simulink model "Noa_Nofusion_backup"  (R2020b)
settings: Solver=FixedStepDiscrete  StartTime=0.0  StopTime=Inf  FixedStep=0.02  RelTol=1e-3
PostLoadFcn:
  | if any(exist('dsrtsu_mdlpostloadfcn', 'file') ~= 0), dsrtsu_mdlpostloadfcn('Execute', bdroot); end
InitFcn:
  | , if any(exist('rtifpga_mdlclblib', 'file') ~= 0), rtifpga_mdlclblib('Init', bdroot); end,
  | , if any(exist('dsmpb_private', 'file') ~= 0), dsmpb_private('dsmpb_mdlclblib', 'Init', bdroot); end,
undefined symbols (not defined in the file): ACC_TimeGap_DecSetSwt, ACC_TimeGap_IncSetSwt, AccelPedalPosn, AccelPedalPosnVldty, AccelPedlPosnDiagc, AccPedalOverride, ACU_ShiftInProgress, ADAS_Posn_CurLane, AESSwtReq, ALC_SwtReq, BrkPedalSts, CC_ACC_CANCEL_OFFSwt, CC_ACC_CRUISE_OFFSwt, CC_ACC_DecSetSpd_SetSwt, CC_ACC_IncSetSpd_ResuSwt, CC_ACCSwtErr, CharSpd_ms, CSA_NODE, CURRENT_GEAR, CurrentGearValid, DiscIntNeverNeededParam, DrvDoorSts, DrvSBR, DrvTrqReqOvld, ECMACCInterface, ECMRespACC, ELKSwtReq, EngLimpHomeSts, EngSpd, EngState, EngState_PHEV, EngTrqMaxActSpd, EngTrqMinAct, EPS_DrvInpTrqVal_HighReslolution, EPS_FailSts, EPS_LKATorqOvrlDlvd, EPS_LKATorqOvrlDlvdVld, EPS_LKATrqOvlDlvdSts, EPS_SteerMod, EPS_TrqSnsrSts, EQ4_APPINFO, EQ4_LA_ELEM, EQ4_LA_HDR, EQ4_LAP_ELEM, EQ4_LAP_HDR, EQ4_LH_ELEM, EQ4_LH_HDR, EQ4_LRE_ELEM, EQ4_LRE_HDR, ESS_PedSwtReq, ESS_VehSwtReq, FFogLmpSts_F_Pbox, FLWheelDriveDirection, FLWheelSpd, FrntWiprSwtSts, FrntWshrSwtSts, FRWheelDriveDirection, FRWheelSpd, HazardLmpSwtSts, HCU_AccelPedalPosn_Diag ... (+152)
libraries: simulink x117, dsmpblib x30
(part 8 of 11)

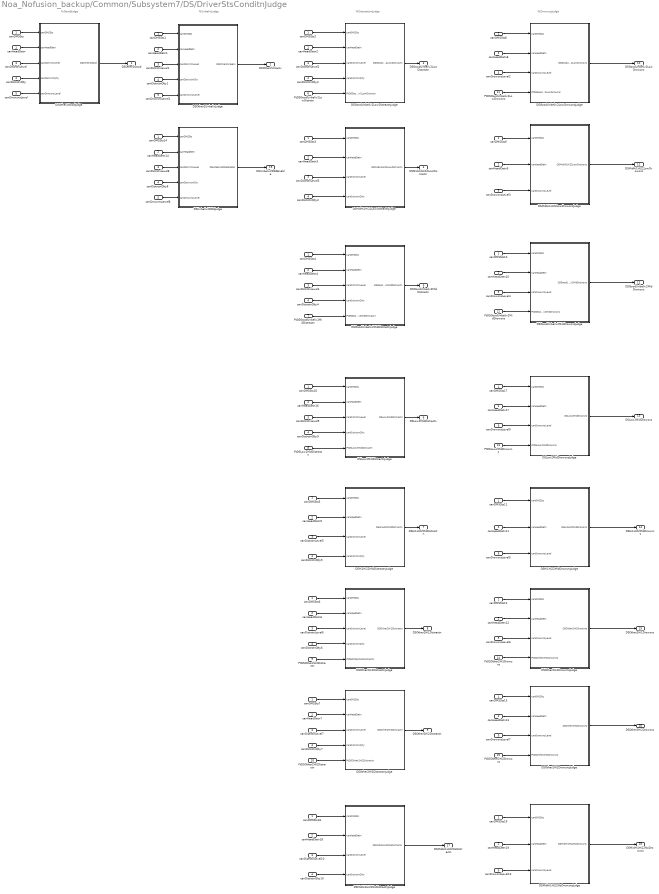
== system Noa_Nofusion_backup/Common/Subsystem7/DS/DriverStsConditnJudge ==
  note: %GoodJudge
  note: %UnbelivJudge
  note: %DistractionJudge
  note: %DrowsnsJudge
  canDMSSts : Inport
  canHeadDetn : Inport  Port=2
  canDistrctnLevel : Inport  Port=3
  canDistrctnQlty : Inport  Port=4
  canDrowsnsLevel : Inport  Port=5
  PtDSGoodUnbeliv2LowDistrctn : Inport  Port=6
  PtDSGoodUnbeliv2MidDistractn : Inport  Port=7
  PtDSLow2MidDistractn : Inport  Port=8
  PtDSOther2Hi1Distractn : Inport  Port=9
  PtDSOther2Hi2Distractn : Inport  Port=10
  PtDSGoodUnbeliv2LowDrowsns : Inport  Port=11
  PtDSGoodUnbeliv2MidDrowsns : Inport  Port=12
  PtDSLow2MidDrowsns : Inport  Port=13
  PtDSOther2Hi1Drowsns : Inport  Port=14
  PtDSOther2Hi2Drowsns : Inport  Port=15
  DSGoodUnbeliv2LowDistractnJudge : Subsystem
  DSGoodUnbeliv2LowDrowsnsJudge : Subsystem
  DSGoodUnbeliv2MidDistractnJudge : Subsystem
  DSGoodUnbeliv2MidDrowsnsJudge : Subsystem
  DSHi1Hi22MidDistractnJudge : Subsystem
  DSHi1Hi22MidDrowsnsJudge : Subsystem
  DSLow2MidDistractnJudge : Subsystem
  DSLow2MidDrowsnsJudge : Subsystem
  DSMidHi1Hi22LowDistractnJudge : Subsystem
  DSMidHi1Hi22LowDrowsnsJudge : Subsystem
  DSMidHi1Hi22NoDistractnJudge : Subsystem
  DSMidHi1Hi22NoDrowsnsJudge : Subsystem
  DSOther2GoodJudge : Subsystem
  DSOther2Hi1DistractnJudge : Subsystem
  DSOther2Hi1DrowsnsJudge : Subsystem
  DSOther2Hi2DistractnJudge : Subsystem
  DSOther2Hi2DrowsnsJudge : Subsystem
  DSOther2UnbelivJudge : Subsystem
  DSUnbeliv2DDAJudge : Subsystem
  canDMSSts{1..14,16..19} (18 alike) : InportShadow
  canDistrctnLevel{1..10} (10 alike) : InportShadow  Port=3
  canDistrctnQlty{1..10} (10 alike) : InportShadow  Port=4
  canDrowsnsLevel{1..10} (10 alike) : InportShadow  Port=5
  canHeadDetn{1..14,16..19} (18 alike) : InportShadow  Port=2
  DSOther2Good : Outport
  DSOther2Unbeliv : Outport  Port=2
  DSGoodUnbeliv2LowDistractn : Outport  Port=3
  DSMidHi1Hi22LowDistractn : Outport  Port=4
  DSGoodUnbeliv2MidDistractn : Outport  Port=5
  DSLow2MidDistractn : Outport  Port=6
  DSHi1Hi22MidDistractn : Outport  Port=7
  DSOther2Hi1Distractn : Outport  Port=8
  DSOther2Hi2Distractn : Outport  Port=9
  DSGoodUnbeliv2LowDrowsns : Outport  Port=10
  DSMidHi1Hi22LowDrowsns : Outport  Port=11
  DSGoodUnbeliv2MidDrowsns : Outport  Port=12
  DSLow2MidDrowsns : Outport  Port=13
  DSHi1Hi22MidDrowsns : Outport  Port=14
  DSOther2Hi1Drowsns : Outport  Port=15
  DSOther2Hi2Drowsns : Outport  Port=16
  DSMidHi1Hi22NoDistractn : Outport  Port=17
  DSMidHi1Hi22NoDrowsns : Outport  Port=18
  DSUnbeliv2DDAEnable : Outport  Port=19
  wires:
  canDMSSts/1 -> DSOther2GoodJudge/1(canDMSSts)
  DSOther2GoodJudge/1(DSOther2Good) -> DSOther2Good/1
  canHeadDetn/1 -> DSOther2GoodJudge/2(canHeadDetn)
  canDistrctnLevel/1 -> DSOther2GoodJudge/3(canDistrctnLevel)
  canDistrctnQlty/1 -> DSOther2GoodJudge/4(canDistrctnQlty)
  canDrowsnsLevel/1 -> DSOther2GoodJudge/5(canDrowsnsLevel)
  canDMSSts1/1 -> DSOther2UnbelivJudge/1(canDMSSts)
  canHeadDetn1/1 -> DSOther2UnbelivJudge/2(canHeadDetn)
  canDistrctnLevel1/1 -> DSOther2UnbelivJudge/3(canDistrctnLevel)
  canDistrctnQlty1/1 -> DSOther2UnbelivJudge/4(canDistrctnQlty)
  canDrowsnsLevel1/1 -> DSOther2UnbelivJudge/5(canDrowsnsLevel)
  DSOther2UnbelivJudge/1(DSOther2Unbeliv) -> DSOther2Unbeliv/1
  DSGoodUnbeliv2LowDistractnJudge/1(DSGoodUnbeliv2LowDistractn) -> DSGoodUnbeliv2LowDistractn/1
  canDMSSts2/1 -> DSGoodUnbeliv2LowDistractnJudge/1(canDMSSts)
  canHeadDetn2/1 -> DSGoodUnbeliv2LowDistractnJudge/2(canHeadDetn)
  canDistrctnLevel2/1 -> DSGoodUnbeliv2LowDistractnJudge/3(canDistrctnLevel)
  canDistrctnQlty2/1 -> DSGoodUnbeliv2LowDistractnJudge/4(canDistrctnQlty)
  canDMSSts3/1 -> DSMidHi1Hi22LowDistractnJudge/1(canDMSSts)
  canHeadDetn3/1 -> DSMidHi1Hi22LowDistractnJudge/2(canHeadDetn)
  canDistrctnLevel3/1 -> DSMidHi1Hi22LowDistractnJudge/3(canDistrctnLevel)
  canDistrctnQlty3/1 -> DSMidHi1Hi22LowDistractnJudge/4(canDistrctnQlty)
  DSMidHi1Hi22LowDistractnJudge/1(DSMidHi1Hi22LowDistractn) -> DSMidHi1Hi22LowDistractn/1
  canDMSSts4/1 -> DSGoodUnbeliv2MidDistractnJudge/1(canDMSSts)
  canHeadDetn4/1 -> DSGoodUnbeliv2MidDistractnJudge/2(canHeadDetn)
  canDistrctnLevel4/1 -> DSGoodUnbeliv2MidDistractnJudge/3(canDistrctnLevel)
  canDistrctnQlty4/1 -> DSGoodUnbeliv2MidDistractnJudge/4(canDistrctnQlty)
  DSGoodUnbeliv2MidDistractnJudge/1(DSGoodUnbeliv2MidDistractn) -> DSGoodUnbeliv2MidDistractn/1
  canDMSSts5/1 -> DSHi1Hi22MidDistractnJudge/1(canDMSSts)
  canHeadDetn5/1 -> DSHi1Hi22MidDistractnJudge/2(canHeadDetn)
  canDistrctnLevel5/1 -> DSHi1Hi22MidDistractnJudge/3(canDistrctnLevel)
  canDistrctnQlty5/1 -> DSHi1Hi22MidDistractnJudge/4(canDistrctnQlty)
  DSHi1Hi22MidDistractnJudge/1(DSHi1Hi22MidDistractn) -> DSHi1Hi22MidDistractn/1
  DSOther2Hi1DistractnJudge/1(DSOther2Hi1Distractn) -> DSOther2Hi1Distractn/1
  canDMSSts6/1 -> DSOther2Hi1DistractnJudge/1(canDMSSts)
  canHeadDetn6/1 -> DSOther2Hi1DistractnJudge/2(canHeadDetn)
  canDistrctnLevel6/1 -> DSOther2Hi1DistractnJudge/3(canDistrctnLevel)
  canDistrctnQlty6/1 -> DSOther2Hi1DistractnJudge/4(canDistrctnQlty)
  DSOther2Hi2DistractnJudge/1(DSOther2Hi2Distractn) -> DSOther2Hi2Distractn/1
  canDMSSts7/1 -> DSOther2Hi2DistractnJudge/1(canDMSSts)
  canHeadDetn7/1 -> DSOther2Hi2DistractnJudge/2(canHeadDetn)
  canDistrctnLevel7/1 -> DSOther2Hi2DistractnJudge/3(canDistrctnLevel)
  canDistrctnQlty7/1 -> DSOther2Hi2DistractnJudge/4(canDistrctnQlty)
  DSGoodUnbeliv2LowDrowsnsJudge/1(DSGoodUnbeliv2LowDrowsns) -> DSGoodUnbeliv2LowDrowsns/1
  canDMSSts8/1 -> DSGoodUnbeliv2LowDrowsnsJudge/1(canDMSSts)
  canHeadDetn8/1 -> DSGoodUnbeliv2LowDrowsnsJudge/2(canHeadDetn)
  canDrowsnsLevel2/1 -> DSGoodUnbeliv2LowDrowsnsJudge/3(canDrowsnsLevel)
  DSMidHi1Hi22LowDrowsnsJudge/1(DSMidHi1Hi22LowDrowsns) -> DSMidHi1Hi22LowDrowsns/1
  canDMSSts9/1 -> DSMidHi1Hi22LowDrowsnsJudge/1(canDMSSts)
  canHeadDetn9/1 -> DSMidHi1Hi22LowDrowsnsJudge/2(canHeadDetn)
  canDrowsnsLevel3/1 -> DSMidHi1Hi22LowDrowsnsJudge/3(canDrowsnsLevel)
  canDMSSts10/1 -> DSGoodUnbeliv2MidDrowsnsJudge/1(canDMSSts)
  canHeadDetn10/1 -> DSGoodUnbeliv2MidDrowsnsJudge/2(canHeadDetn)
  canDrowsnsLevel4/1 -> DSGoodUnbeliv2MidDrowsnsJudge/3(canDrowsnsLevel)
  DSGoodUnbeliv2MidDrowsnsJudge/1(DSGoodUnbeliv2MidDrowsns) -> DSGoodUnbeliv2MidDrowsns/1
  DSHi1Hi22MidDrowsnsJudge/1(DSHi1Hi22MidDrowsns) -> DSHi1Hi22MidDrowsns/1
  canDrowsnsLevel5/1 -> DSHi1Hi22MidDrowsnsJudge/3(canDrowsnsLevel)
  canHeadDetn11/1 -> DSHi1Hi22MidDrowsnsJudge/2(canHeadDetn)
  canDMSSts11/1 -> DSHi1Hi22MidDrowsnsJudge/1(canDMSSts)
  canDMSSts12/1 -> DSOther2Hi1DrowsnsJudge/1(canDMSSts)
  canHeadDetn12/1 -> DSOther2Hi1DrowsnsJudge/2(canHeadDetn)
  canDrowsnsLevel6/1 -> DSOther2Hi1DrowsnsJudge/3(canDrowsnsLevel)
  DSOther2Hi1DrowsnsJudge/1(DSOther2Hi1Drowsns) -> DSOther2Hi1Drowsns/1
  canDrowsnsLevel7/1 -> DSOther2Hi2DrowsnsJudge/3(canDrowsnsLevel)
  canHeadDetn13/1 -> DSOther2Hi2DrowsnsJudge/2(canHeadDetn)
  canDMSSts13/1 -> DSOther2Hi2DrowsnsJudge/1(canDMSSts)
  DSOther2Hi2DrowsnsJudge/1(DSOther2Hi2Drowsns) -> DSOther2Hi2Drowsns/1
  DSLow2MidDistractnJudge/1(DSLow2MidDistractn) -> DSLow2MidDistractn/1
  canDistrctnQlty9/1 -> DSLow2MidDistractnJudge/4(canDistrctnQlty)
  canDistrctnLevel9/1 -> DSLow2MidDistractnJudge/3(canDistrctnLevel)
  canHeadDetn16/1 -> DSLow2MidDistractnJudge/2(canHeadDetn)
  canDMSSts16/1 -> DSLow2MidDistractnJudge/1(canDMSSts)
  canDrowsnsLevel9/1 -> DSLow2MidDrowsnsJudge/3(canDrowsnsLevel)
  canHeadDetn17/1 -> DSLow2MidDrowsnsJudge/2(canHeadDetn)
  canDMSSts17/1 -> DSLow2MidDrowsnsJudge/1(canDMSSts)
  DSLow2MidDrowsnsJudge/1(DSLow2MidDrowsns) -> DSLow2MidDrowsns/1
  canDistrctnQlty10/1 -> DSMidHi1Hi22NoDistractnJudge/4(canDistrctnQlty)
  canDistrctnLevel10/1 -> DSMidHi1Hi22NoDistractnJudge/3(canDistrctnLevel)
  canHeadDetn18/1 -> DSMidHi1Hi22NoDistractnJudge/2(canHeadDetn)
  canDMSSts18/1 -> DSMidHi1Hi22NoDistractnJudge/1(canDMSSts)
  DSMidHi1Hi22NoDistractnJudge/1(DSMidHi1Hi22NoDistractn) -> DSMidHi1Hi22NoDistractn/1
  canDrowsnsLevel10/1 -> DSMidHi1Hi22NoDrowsnsJudge/3(canDrowsnsLevel)
  canHeadDetn19/1 -> DSMidHi1Hi22NoDrowsnsJudge/2(canHeadDetn)
  canDMSSts19/1 -> DSMidHi1Hi22NoDrowsnsJudge/1(canDMSSts)
  DSMidHi1Hi22NoDrowsnsJudge/1(DSMidHi1Hi22NoDrowsns) -> DSMidHi1Hi22NoDrowsns/1
  canDrowsnsLevel8/1 -> DSUnbeliv2DDAJudge/5(canDrowsnsLevel)
  canDistrctnQlty8/1 -> DSUnbeliv2DDAJudge/4(canDistrctnQlty)
  canDistrctnLevel8/1 -> DSUnbeliv2DDAJudge/3(canDistrctnLevel)
  canHeadDetn14/1 -> DSUnbeliv2DDAJudge/2(canHeadDetn)
  canDMSSts14/1 -> DSUnbeliv2DDAJudge/1(canDMSSts)
  DSUnbeliv2DDAJudge/1(DSUnbeliv2DDAEnable) -> DSUnbeliv2DDAEnable/1
  PtDSGoodUnbeliv2LowDistrctn/1 -> DSGoodUnbeliv2LowDistractnJudge/5(PtDSGoodUnbeliv2LowDistrctn)
  PtDSGoodUnbeliv2MidDistractn/1 -> DSGoodUnbeliv2MidDistractnJudge/5(PtDSGoodUnbeliv2MidDistractn)
  PtDSLow2MidDistractn/1 -> DSLow2MidDistractnJudge/5(PtDSLow2MidDistractn)
  PtDSOther2Hi1Distractn/1 -> DSOther2Hi1DistractnJudge/5(PtDSOther2Hi1Distractn)
  PtDSOther2Hi2Distractn/1 -> DSOther2Hi2DistractnJudge/5(PtDSOther2Hi2Distractn)
  PtDSGoodUnbeliv2LowDrowsns/1 -> DSGoodUnbeliv2LowDrowsnsJudge/4(PtDSGoodUnbeliv2LowDrowsns)
  PtDSGoodUnbeliv2MidDrowsns/1 -> DSGoodUnbeliv2MidDrowsnsJudge/4(PtDSGoodUnbeliv2MidDrowsns)
  PtDSLow2MidDrowsns/1 -> DSLow2MidDrowsnsJudge/4(PtDSLow2MidDrowsns)
  PtDSOther2Hi1Drowsns/1 -> DSOther2Hi1DrowsnsJudge/4(PtDSOther2Hi1Drowsns)
  PtDSOther2Hi2Drowsns/1 -> DSOther2Hi2DrowsnsJudge/4(PtDSOther2Hi2Drowsns)

== system Noa_Nofusion_backup/Subsystem2/ACCOSM/HWA_Task100ms1/OTL1 ==
  vRef : Inport
  tCycle : Inport  Port=2
  tSameHandle : Inport  Port=3
  CutIn : Inport  Port=4
  P0Dx : Inport  Port=5
  P0Dy : Inport  Port=6
  EgoDDeltaX : Inport  Port=7
  EgoDDeltaY : Inport  Port=8
  EgoCosOfPsi : Inport  Port=9
  EgoSinOfPsi : Inport  Port=10
  Memory31 : Memory  InitialCondition=zeros(24,1)  InheritSampleTime=on
  Memory32 : Memory  InitialCondition=zeros(24,1)  InheritSampleTime=on
  Memory33 : Memory  InitialCondition=uint8(0)  InheritSampleTime=on
  P0TrajHistCalc01 : MATLAB Function  TreatAsAtomicUnit=on
  P0TrajHistCalc1 : MATLAB Function  TreatAsAtomicUnit=on
  Terminator : Terminator
  Terminator1 : Terminator
  Terminator2 : Terminator
  LineValid : Outport
  a : Outport  Port=2
  b : Outport  Port=3
  c : Outport  Port=4
  d : Outport  Port=5
  dxMin : Outport  Port=6
  dxMax : Outport  Port=7
  wires:
  vRef/1 -> P0TrajHistCalc01/1(vRef)
  CutIn/1 -> P0TrajHistCalc01/4(CutIn)
  P0TrajHistCalc1/8(d) -> d/1
  P0TrajHistCalc1/10(dxMax) -> dxMax/1
  P0TrajHistCalc1/9(dxMin) -> dxMin/1
  P0TrajHistCalc1/7(c) -> c/1
  P0TrajHistCalc1/6(b) -> b/1
  P0TrajHistCalc1/5(a) -> a/1
  P0TrajHistCalc1/4(LineValid) -> LineValid/1
  P0TrajHistCalc1/3(P0TrajHistDyv) -> Terminator2/1
  P0TrajHistCalc1/2(P0TrajHistDxv) -> Terminator1/1
  P0TrajHistCalc1/1(P0TrajHistNum) -> Terminator/1
  P0Dy/1 -> P0TrajHistCalc01/6(P0Dy)
  P0Dx/1 -> P0TrajHistCalc01/5(P0Dx)
  tSameHandle/1 -> P0TrajHistCalc01/3(tSameHandle)
  EgoCosOfPsi/1 -> P0TrajHistCalc01/9(EgoCosOfPsi)
  tCycle/1 -> P0TrajHistCalc01/2(tCycle)
  Memory31/1 -> P0TrajHistCalc01/13(P0TrajHistDyvK1)
  EgoDDeltaY/1 -> P0TrajHistCalc01/8(EgoDDeltaY)
  P0TrajHistCalc01/2(P0TrajHistDxv) -> Memory32/1, P0TrajHistCalc1/2(P0TrajHistDxv1)
  Memory32/1 -> P0TrajHistCalc01/12(P0TrajHistDxvK1)
  P0TrajHistCalc01/1(P0TrajHistNum) -> Memory33/1, P0TrajHistCalc1/1(P0TrajHistNum1)
  EgoSinOfPsi/1 -> P0TrajHistCalc01/10(EgoSinOfPsi)
  Memory33/1 -> P0TrajHistCalc01/11(P0TrajHistNumK1)
  P0TrajHistCalc01/3(P0TrajHistDyv) -> Memory31/1, P0TrajHistCalc1/3(P0TrajHistDyv1)
  EgoDDeltaX/1 -> P0TrajHistCalc01/7(EgoDDeltaX)

== system Noa_Nofusion_backup/Subsystem2/ACCOSM/HWA_Task100ms1/Trajectory ==
  Kap : Inport
  VxvRef : Inport  Port=2
  AlpSideSlipAngle : Inport  Port=3
  ObjValid : Inport  Port=4
  ObjDx : Inport  Port=5
  ObjDy : Inport  Port=6
  ObjClass : Inport  Port=7
  ObjCntAlive : Inport  Port=8
  Terminator{1,3..10} (9 alike) : Terminator
  Trajectory : Subsystem  mask{ObjNum=15, TrajNum=10, BufNum=24}
      mask prompts: ObjNum "ObjectNumber"; TrajNum "TrajectoryNumber"; BufNum "BufferNumber"
  Out8 : Outport
  Out9 : Outport  Port=2
  Out10 : Outport  Port=3
  Out11 : Outport  Port=4
  Out12 : Outport  Port=5
  Out13 : Outport  Port=6
  EgoMove : Outport  Port=7
  wires:
  Trajectory/16(EgoMove) -> EgoMove/1
  Trajectory/11(TrajHistBufferBValid) -> Out11/1
  Trajectory/12(TrajHistBufferDxv) -> Out12/1
  Trajectory/13(TrajHistBufferDyv) -> Out13/1
  ObjValid/1 -> Trajectory/4(ObjValid)
  ObjDx/1 -> Trajectory/5(ObjectDx)
  ObjDy/1 -> Trajectory/6(ObjectDy)
  ObjClass/1 -> Trajectory/7(ObjectClass)
  ObjCntAlive/1 -> Trajectory/8(ObjectCntAlive)
  Kap/1 -> Trajectory/1(KapTraj)
  Trajectory/8(TrajHistBufferBTrajEnd) -> Out8/1
  Trajectory/2(EgoTrajHistDxv) -> Terminator4/1
  Trajectory/5(ObjPrio) -> Terminator8/1
  Trajectory/1(EgoTrajHistCurrentIndex) -> Terminator3/1
  AlpSideSlipAngle/1 -> Trajectory/3(AlpSideSlipAngle)
  Trajectory/7(TrajUsed) -> Terminator9/1
  Trajectory/10(TrajCurrentIndex) -> Out10/1
  Trajectory/6(ObjMatrix) -> Terminator10/1
  Trajectory/4(EgoTrajHistTTimeStamp) -> Terminator7/1
  VxvRef/1 -> Trajectory/2(VxvRef)
  Trajectory/3(EgoTrajHistDyv) -> Terminator5/1
  Trajectory/9(ObjTrajNumber) -> Out9/1
  Trajectory/14(TrajHistBufferTTimeStamp) -> Terminator6/1
  Trajectory/15(TrajHistBufferClass) -> Terminator1/1

== system Noa_Nofusion_backup/Subsystem2/ACCOSM/HWA_Task100ms1/VxVy ==
  VxvRef : Inport
  Kap : Inport  Port=2
  VxG : Inport  Port=3
  VyG : Inport  Port=4
  Constant2 : Constant  Value=P_Global_EQ2RearAxisX_m  OutDataTypeStr=single
  Constant4 : Constant  Value=SideSlipAnglefactor  OutDataTypeStr=single
  Divide11 : Product
  Divide3 : Product  Inputs=3
  Divide4 : Product
  Divide5 : Product
  Gain10 : Gain  Gain=-1
  Gain9 : Gain  Gain=-1
  Sum1 : Sum  Inputs=+-
  Sum10 : Sum  Inputs=+-|
  Sum11 : Sum  Inputs=|-+
  Trigonometric Function : Trigonometry  Operator=atan  OutputSignalType=real
  Trigonometric Function1 : Trigonometry  Operator=cos
  Trigonometric Function2 : Trigonometry
  Vx : Outport
  Vy : Outport  Port=2
  wires:
  VxvRef/1 -> Divide3/2, Divide11/1, Divide5/1, Divide3/3
  Constant4/1 -> Divide3/1
  Trigonometric Function/1 -> Gain9/1
  Divide11/1 -> Sum11/1
  Constant2/1 -> Sum1/1
  Trigonometric Function1/1 -> Divide5/2
  Divide4/1 -> Trigonometric Function/1
  Divide5/1 -> Sum10/2
  Gain10/1 -> Trigonometric Function1/1, Trigonometric Function2/1
  Divide3/1 -> Sum1/2
  [IFVMoveAngle] -> Gain10/1
  Trigonometric Function2/1 -> Divide11/2
  Sum1/1 -> Divide4/1
  Gain9/1 -> [IFVMoveAngle]
  VxG/1 -> Sum10/1
  Sum11/1 -> Vy/1  "Vy"
  Sum10/1 -> Vx/1  "Vx"
  VyG/1 -> Sum11/2
  Kap/1 -> Divide4/2

== system Noa_Nofusion_backup/Subsystem2/ACCOSM/ObjMatrixTransit/Subsystem ==
  Count : Inport
  <EQ4_OBJ_ELEM> : Inport  Port=2
  Bus Creator : BusCreator  Inputs=12
  Bus Selector : BusSelector  OutputSignals=id,BrakeLight,classification,LatDis,AbsLatVel,AbsLongAcc,LongDis,AbsLongVel,width,Age,motionSts
  For Each Subsystem : Subsystem  TreatAsAtomicUnit=on
  For Iterator Subsystem : Subsystem  Commented=on  TreatAsAtomicUnit=on
  MATLAB Function1 : MATLAB Function  TreatAsAtomicUnit=on
  Obj : Stateflow chart  Commented=on  TreatAsAtomicUnit=on
  Terminator : Terminator
  Terminator1 : Terminator
  Unit Delay1 : UnitDelay  SampleTime=-1  HasFrameUpgradeWarning=on
  ObjID : Outport
  ObjValid : Outport  Port=2
  ObjBrakeLightIndic : Outport  Port=3
  ObjClassification : Outport  Port=4
  ObjLatPos : Outport  Port=5
  ObjLatVel : Outport  Port=6
  ObjLongAccel : Outport  Port=7
  ObjLongVel : Outport  Port=8
  ObjWidth : Outport  Port=9
  ObjCnt : Outport  Port=10
  ObjMoveSts : Outport  Port=11
  ObjLongPos : Outport  Port=12
  P : Outport  Port=13
  wires:
  MATLAB Function1/10(ObjCnt) -> ObjCnt/1
  MATLAB Function1/9(ObjWidth) -> ObjWidth/1
  MATLAB Function1/8(ObjLongVel) -> ObjLongVel/1
  MATLAB Function1/3(ObjBrakeLightIndic) -> ObjBrakeLightIndic/1
  MATLAB Function1/6(ObjLatVel) -> ObjLatVel/1
  MATLAB Function1/2(ObjValid) -> ObjValid/1
  <EQ4_OBJ_ELEM>/1 -> For Each Subsystem/1(<EQ4_OBJ_ELEM>)
  Unit Delay1/1 -> MATLAB Function1/13(ObjIDK1)
  Bus Selector/1 -> MATLAB Function1/2(ID)  "<id>"
  Bus Selector/2 -> MATLAB Function1/3(BrakeLight_b)  "<BrakeLight>"
  MATLAB Function1/1(P) -> P/1
  MATLAB Function1/12(ObjLongPos) -> ObjLongPos/1
  Bus Selector/11 -> MATLAB Function1/12(MotionSts)  "<motionSts>"
  MATLAB Function1/11(ObjMoveSts) -> ObjMoveSts/1
  Bus Selector/4 -> MATLAB Function1/5(LatDis)  "<LatDis>"
  Bus Selector/6 -> MATLAB Function1/7(LongAccel)  "<AbsLongAcc>"
  Bus Selector/5 -> MATLAB Function1/6(LatVel)  "<AbsLatVel>"
  Bus Selector/9 -> MATLAB Function1/10(Width)  "<width>"
  Bus Selector/7 -> MATLAB Function1/8(LongDis)  "<LongDis>"
  For Each Subsystem/2(confidence) -> Bus Creator/2  "confidence"
  For Each Subsystem/11(Age) -> Bus Creator/11  "Age"
  For Each Subsystem/1(id) -> Bus Creator/1  "id"
  Bus Selector/3 -> MATLAB Function1/4(Class)  "<classification>"
  Bus Selector/8 -> MATLAB Function1/9(LongVel)  "<AbsLongVel>"
  For Each Subsystem/3(classification) -> Bus Creator/3  "classification"
  Bus Selector/10 -> MATLAB Function1/11(Age)  "<Age>"
  For Each Subsystem/5(LongDis) -> Bus Creator/5  "LongDis"
  For Each Subsystem/9(AbsLatVel) -> Bus Creator/9  "AbsLatVel"
  For Each Subsystem/13(motionCategory) -> Terminator/1
  For Each Subsystem/4(width) -> Bus Creator/4  "width"
  For Each Subsystem/8(AbsLongVel) -> Bus Creator/8  "AbsLongVel"
  Count/1 -> MATLAB Function1/1(Count)
  For Each Subsystem/14(motionOrientation) -> Terminator1/1
  MATLAB Function1/7(ObjLongAccel) -> ObjLongAccel/1
  MATLAB Function1/4(ObjClassification) -> ObjClassification/1
  For Each Subsystem/12(motionSts) -> Bus Creator/12  "motionSts"
  For Each Subsystem/7(AbsLongAcc) -> Bus Creator/7  "AbsLongAcc"
  MATLAB Function1/5(ObjLatPos) -> ObjLatPos/1
  For Each Subsystem/10(BrakeLight) -> Bus Creator/10  "BrakeLight"
  MATLAB Function1/13(ObjID) -> Unit Delay1/1, ObjID/1  "ObjBrakeLightIndic"
  Bus Creator/1 -> Bus Selector/1
  For Each Subsystem/6(LatDis) -> Bus Creator/6  "LatDis"

== system Noa_Nofusion_backup/Common/Subsystem7/DS/DriverStsConditnJudge/DSGoodUnbeliv2LowDistractnJudge ==
  note: %Note
      | Conditions of distraction state from Good∥Unbelievable to Low as follow:
      | DMSSts_ACC is 0x02: Active
      | && HeadDetn is 0x01: Yes
      | && DistrctnLevel_ACC is 0x01: Low level distraction
      | && DistrctnQlty_ACC≥ 85%
      | && During time≥1s(adjustable)
  canDMSSts : Inport
  canHeadDetn : Inport  Port=2
  canDistrctnLevel : Inport  Port=3
  canDistrctnQlty : Inport  Port=4
  PtDSGoodUnbeliv2LowDistrctn : Inport  Port=5
  Compare To Constant : simulink/Logic and Bit Operations/Compare To Constant  relop===  const=2  OutDataTypeStr=boolean
  Compare To Constant1 : simulink/Logic and Bit Operations/Compare To Constant  relop===  const=1  OutDataTypeStr=boolean
  Compare To Constant2 : simulink/Logic and Bit Operations/Compare To Constant  relop===  const=1  OutDataTypeStr=boolean
  Compare To Constant4 : simulink/Logic and Bit Operations/Compare To Constant  relop=>=  const=85  OutDataTypeStr=boolean
  Compare To Constant8 : simulink/Logic and Bit Operations/Compare To Constant  relop=<=  const=100  OutDataTypeStr=boolean
  Data Type Conversion : DataTypeConversion  OutDataTypeStr=single
  Logical Operator : Logic  Inputs=5  AllPortsSameDT=off  OutDataTypeStr=boolean
  Relational Operator : RelationalOperator  OutDataTypeStr=boolean  RndMeth=Simplest
  counter : DiscreteIntegrator  ExternalReset=either  SampleTime=-1  LimitOutput=on  UpperSaturationLimit=10  LowerSaturationLimit=-10  ICPrevOutput=DiscIntNeverNeededParam  ICPrevScaledInput=DiscIntNeverNeededParam
  DSGoodUnbeliv2LowDistractn : Outport
  wires:
  canDMSSts/1 -> Compare To Constant/1
  canHeadDetn/1 -> Compare To Constant1/1
  canDistrctnLevel/1 -> Compare To Constant2/1
  Logical Operator/1 -> Data Type Conversion/1
  counter/1 -> Relational Operator/1
  canDistrctnQlty/1 -> Compare To Constant8/1, Compare To Constant4/1
  Compare To Constant1/1 -> Logical Operator/2
  Compare To Constant/1 -> Logical Operator/1
  Compare To Constant2/1 -> Logical Operator/3
  Compare To Constant4/1 -> Logical Operator/4
  Compare To Constant8/1 -> Logical Operator/5
  Relational Operator/1 -> DSGoodUnbeliv2LowDistractn/1
  PtDSGoodUnbeliv2LowDistrctn/1 -> Relational Operator/2
  Data Type Conversion/1 -> counter/2, counter/1

== system Noa_Nofusion_backup/Common/Subsystem7/DS/DriverStsConditnJudge/DSGoodUnbeliv2LowDrowsnsJudge ==
  note: %Note
      | Conditions of drowsns state from Good∥Unbelievable to Low as follow:
      | DMSSts_ACC is 0x02: Active
      | && HeadDetn is 0x01: Yes
      | && DrowsnsLevel_ACC is 0x1: Low level Drowsiness
      | && DrowsnsQlty_ACC≥85%
      | && During time≥3s(adjustable)
  canDMSSts : Inport
  canHeadDetn : Inport  Port=2
  canDrowsnsLevel : Inport  Port=3
  PtDSGoodUnbeliv2LowDrowsns : Inport  Port=4
  Compare To Constant : simulink/Logic and Bit Operations/Compare To Constant  relop===  const=2  OutDataTypeStr=boolean
  Compare To Constant1 : simulink/Logic and Bit Operations/Compare To Constant  relop===  const=1  OutDataTypeStr=boolean
  Compare To Constant2 : simulink/Logic and Bit Operations/Compare To Constant  relop===  const=1  OutDataTypeStr=boolean
  Data Type Conversion : DataTypeConversion  OutDataTypeStr=single
  Logical Operator : Logic  Inputs=3  AllPortsSameDT=off  OutDataTypeStr=boolean
  Relational Operator : RelationalOperator  OutDataTypeStr=boolean  RndMeth=Simplest
  counter : DiscreteIntegrator  ExternalReset=either  SampleTime=-1  LimitOutput=on  UpperSaturationLimit=10  LowerSaturationLimit=-10  ICPrevOutput=DiscIntNeverNeededParam  ICPrevScaledInput=DiscIntNeverNeededParam
  DSGoodUnbeliv2LowDrowsns : Outport
  wires:
  Relational Operator/1 -> DSGoodUnbeliv2LowDrowsns/1
  Compare To Constant2/1 -> Logical Operator/3
  Compare To Constant/1 -> Logical Operator/1
  Compare To Constant1/1 -> Logical Operator/2
  counter/1 -> Relational Operator/1
  Logical Operator/1 -> Data Type Conversion/1
  canDrowsnsLevel/1 -> Compare To Constant2/1
  canHeadDetn/1 -> Compare To Constant1/1
  canDMSSts/1 -> Compare To Constant/1
  PtDSGoodUnbeliv2LowDrowsns/1 -> Relational Operator/2
  Data Type Conversion/1 -> counter/1, counter/2

== system Noa_Nofusion_backup/Common/Subsystem7/DS/DriverStsConditnJudge/DSGoodUnbeliv2MidDistractnJudge ==
  note: %Note
      | Conditions of distraction state from Good∥Unbelievable to Middle as follow:
      | DMSSts_ACC is 0x02: Active
      | && HeadDetn is 0x01: Yes
      | && DistrctnLevel_ACC is 0x02: Middle level distraction
      | && DistrctnQlty_ACC≥ 85%
      | && During time≥2s(adjustable)
  canDMSSts : Inport
  canHeadDetn : Inport  Port=2
  canDistrctnLevel : Inport  Port=3
  canDistrctnQlty : Inport  Port=4
  PtDSGoodUnbeliv2MidDistractn : Inport  Port=5
  Compare To Constant : simulink/Logic and Bit Operations/Compare To Constant  relop===  const=2  OutDataTypeStr=boolean
  Compare To Constant1 : simulink/Logic and Bit Operations/Compare To Constant  relop===  const=1  OutDataTypeStr=boolean
  Compare To Constant2 : simulink/Logic and Bit Operations/Compare To Constant  relop===  const=2  OutDataTypeStr=boolean
  Compare To Constant4 : simulink/Logic and Bit Operations/Compare To Constant  relop=>=  const=85  OutDataTypeStr=boolean
  Compare To Constant8 : simulink/Logic and Bit Operations/Compare To Constant  relop=<=  const=100  OutDataTypeStr=boolean
  Data Type Conversion : DataTypeConversion  OutDataTypeStr=single
  Logical Operator : Logic  Inputs=5  AllPortsSameDT=off  OutDataTypeStr=boolean
  Relational Operator : RelationalOperator  OutDataTypeStr=boolean  RndMeth=Simplest
  counter : DiscreteIntegrator  ExternalReset=either  SampleTime=-1  LimitOutput=on  UpperSaturationLimit=10  LowerSaturationLimit=-10  ICPrevOutput=DiscIntNeverNeededParam  ICPrevScaledInput=DiscIntNeverNeededParam
  DSGoodUnbeliv2MidDistractn : Outport
  wires:
  canDMSSts/1 -> Compare To Constant/1
  canHeadDetn/1 -> Compare To Constant1/1
  canDistrctnLevel/1 -> Compare To Constant2/1
  Logical Operator/1 -> Data Type Conversion/1
  canDistrctnQlty/1 -> Compare To Constant8/1, Compare To Constant4/1
  Compare To Constant1/1 -> Logical Operator/2
  Compare To Constant/1 -> Logical Operator/1
  Compare To Constant2/1 -> Logical Operator/3
  Compare To Constant4/1 -> Logical Operator/4
  Compare To Constant8/1 -> Logical Operator/5
  Relational Operator/1 -> DSGoodUnbeliv2MidDistractn/1
  PtDSGoodUnbeliv2MidDistractn/1 -> Relational Operator/2
  counter/1 -> Relational Operator/1
  Data Type Conversion/1 -> counter/2, counter/1

== system Noa_Nofusion_backup/Common/Subsystem7/DS/DriverStsConditnJudge/DSGoodUnbeliv2MidDrowsnsJudge ==
  note: %Note
      | Conditions of drowsns state from Good∥Unbelievable to Middle as follow:
      | DMSSts_ACC is 0x02: Active
      | && HeadDetn is 0x01: Yes
      | && DrowsnsLevel_ACC is 0x2: Middle level Drowsiness
      | && DrowsnsQlty_ACC≥85%
      | && During time≥3s(adjustable)
  canDMSSts : Inport
  canHeadDetn : Inport  Port=2
  canDrowsnsLevel : Inport  Port=3
  PtDSGoodUnbeliv2MidDrowsns : Inport  Port=4
  Compare To Constant : simulink/Logic and Bit Operations/Compare To Constant  relop===  const=2  OutDataTypeStr=boolean
  Compare To Constant1 : simulink/Logic and Bit Operations/Compare To Constant  relop===  const=1  OutDataTypeStr=boolean
  Compare To Constant2 : simulink/Logic and Bit Operations/Compare To Constant  relop===  const=2  OutDataTypeStr=boolean
  Data Type Conversion : DataTypeConversion  OutDataTypeStr=single
  Logical Operator : Logic  Inputs=3  AllPortsSameDT=off  OutDataTypeStr=boolean
  Relational Operator : RelationalOperator  OutDataTypeStr=boolean  RndMeth=Simplest
  counter : DiscreteIntegrator  ExternalReset=either  SampleTime=-1  LimitOutput=on  UpperSaturationLimit=10  LowerSaturationLimit=-10  ICPrevOutput=DiscIntNeverNeededParam  ICPrevScaledInput=DiscIntNeverNeededParam
  DSGoodUnbeliv2MidDrowsns : Outport
  wires:
  Compare To Constant2/1 -> Logical Operator/3
  Compare To Constant/1 -> Logical Operator/1
  Compare To Constant1/1 -> Logical Operator/2
  Relational Operator/1 -> DSGoodUnbeliv2MidDrowsns/1
  counter/1 -> Relational Operator/1
  Logical Operator/1 -> Data Type Conversion/1
  canDrowsnsLevel/1 -> Compare To Constant2/1
  canHeadDetn/1 -> Compare To Constant1/1
  canDMSSts/1 -> Compare To Constant/1
  PtDSGoodUnbeliv2MidDrowsns/1 -> Relational Operator/2
  Data Type Conversion/1 -> counter/2, counter/1

== system Noa_Nofusion_backup/Common/Subsystem7/DS/DriverStsConditnJudge/DSHi1Hi22MidDistractnJudge ==
  note: %Note
      | Conditions of distraction state from High Level 1∥High Level 2 to Middle as follow:
      | DMSSts_ACC is 0x02: Active
      | && HeadDetn is 0x01: Yes
      | && DistrctnLevel_ACC is 0x02: Middle level distraction
      | && DistrctnQlty_ACC≥ 85%
      | && During time≥0.5s(adjustable)
  canDMSSts : Inport
  canHeadDetn : Inport  Port=2
  canDistrctnLevel : Inport  Port=3
  canDistrctnQlty : Inport  Port=4
  Compare To Constant : simulink/Logic and Bit Operations/Compare To Constant  relop===  const=2  OutDataTypeStr=boolean
  Compare To Constant1 : simulink/Logic and Bit Operations/Compare To Constant  relop===  const=1  OutDataTypeStr=boolean
  Compare To Constant2 : simulink/Logic and Bit Operations/Compare To Constant  relop===  const=2  OutDataTypeStr=boolean
  Compare To Constant4 : simulink/Logic and Bit Operations/Compare To Constant  relop=>=  const=85  OutDataTypeStr=boolean
  Compare To Constant5 : simulink/Logic and Bit Operations/Compare To Constant  relop=>=  const=0.5  OutDataTypeStr=boolean
  Compare To Constant8 : simulink/Logic and Bit Operations/Compare To Constant  relop=<=  const=100  OutDataTypeStr=boolean
  Data Type Conversion : DataTypeConversion  OutDataTypeStr=single
  Logical Operator : Logic  Inputs=5  AllPortsSameDT=off  OutDataTypeStr=boolean
  counter : DiscreteIntegrator  ExternalReset=either  SampleTime=-1  LimitOutput=on  UpperSaturationLimit=10  LowerSaturationLimit=-10  ICPrevOutput=DiscIntNeverNeededParam  ICPrevScaledInput=DiscIntNeverNeededParam
  DSHi1Hi22MidDistractn : Outport
  wires:
  Compare To Constant5/1 -> DSHi1Hi22MidDistractn/1
  Compare To Constant8/1 -> Logical Operator/5
  Compare To Constant4/1 -> Logical Operator/4
  Compare To Constant2/1 -> Logical Operator/3
  Compare To Constant/1 -> Logical Operator/1
  Compare To Constant1/1 -> Logical Operator/2
  canDistrctnQlty/1 -> Compare To Constant4/1, Compare To Constant8/1
  counter/1 -> Compare To Constant5/1
  Logical Operator/1 -> Data Type Conversion/1
  canDistrctnLevel/1 -> Compare To Constant2/1
  canHeadDetn/1 -> Compare To Constant1/1
  canDMSSts/1 -> Compare To Constant/1
  Data Type Conversion/1 -> counter/2, counter/1

== system Noa_Nofusion_backup/Common/Subsystem7/DS/DriverStsConditnJudge/DSHi1Hi22MidDrowsnsJudge ==
  note: %Note
      | Conditions of drowsns state from High Level 1∥High Level 2 to Middle as follow:
      | DMSSts_ACC is 0x02: Active
      | && HeadDetn is 0x01: Yes
      | && DrowsnsLevel_ACC is 0x2: Middle level Drowsiness
      | && DrowsnsQlty_ACC≥85%
      | && During time≥0.5s(adjustable)
  canDMSSts : Inport
  canHeadDetn : Inport  Port=2
  canDrowsnsLevel : Inport  Port=3
  Compare To Constant : simulink/Logic and Bit Operations/Compare To Constant  relop===  const=2  OutDataTypeStr=boolean
  Compare To Constant1 : simulink/Logic and Bit Operations/Compare To Constant  relop===  const=1  OutDataTypeStr=boolean
  Compare To Constant2 : simulink/Logic and Bit Operations/Compare To Constant  relop===  const=2  OutDataTypeStr=boolean
  Compare To Constant5 : simulink/Logic and Bit Operations/Compare To Constant  relop=>=  const=0.5  OutDataTypeStr=boolean
  Data Type Conversion : DataTypeConversion  OutDataTypeStr=single
  Logical Operator : Logic  Inputs=3  AllPortsSameDT=off  OutDataTypeStr=boolean
  counter : DiscreteIntegrator  ExternalReset=either  SampleTime=-1  LimitOutput=on  UpperSaturationLimit=10  LowerSaturationLimit=-10  ICPrevOutput=DiscIntNeverNeededParam  ICPrevScaledInput=DiscIntNeverNeededParam
  DSHi1Hi22MidDrowsns : Outport
  wires:
  canDMSSts/1 -> Compare To Constant/1
  canHeadDetn/1 -> Compare To Constant1/1
  canDrowsnsLevel/1 -> Compare To Constant2/1
  Logical Operator/1 -> Data Type Conversion/1
  counter/1 -> Compare To Constant5/1
  Compare To Constant1/1 -> Logical Operator/2
  Compare To Constant/1 -> Logical Operator/1
  Compare To Constant2/1 -> Logical Operator/3
  Compare To Constant5/1 -> DSHi1Hi22MidDrowsns/1
  Data Type Conversion/1 -> counter/2, counter/1

== system Noa_Nofusion_backup/Common/Subsystem7/DS/DriverStsConditnJudge/DSLow2MidDistractnJudge ==
  note: %Note
      | Conditions of distraction state from Low to Middle as follow:
      | DMSSts_ACC is 0x02: Active
      | && HeadDetn is 0x01: Yes
      | && DistrctnLevel_ACC is 0x02: Middle level distraction
      | && DistrctnQlty_ACC≥ 85%
      | && During time≥2s(adjustable)
  canDMSSts : Inport
  canHeadDetn : Inport  Port=2
  canDistrctnLevel : Inport  Port=3
  canDistrctnQlty : Inport  Port=4
  PtDSLow2MidDistractn : Inport  Port=5
  Compare To Constant : simulink/Logic and Bit Operations/Compare To Constant  relop===  const=2  OutDataTypeStr=boolean
  Compare To Constant1 : simulink/Logic and Bit Operations/Compare To Constant  relop===  const=1  OutDataTypeStr=boolean
  Compare To Constant2 : simulink/Logic and Bit Operations/Compare To Constant  relop===  const=2  OutDataTypeStr=boolean
  Compare To Constant4 : simulink/Logic and Bit Operations/Compare To Constant  relop=>=  const=85  OutDataTypeStr=boolean
  Compare To Constant8 : simulink/Logic and Bit Operations/Compare To Constant  relop=<=  const=100  OutDataTypeStr=boolean
  Data Type Conversion : DataTypeConversion  OutDataTypeStr=single
  Logical Operator : Logic  Inputs=5  AllPortsSameDT=off  OutDataTypeStr=boolean
  Relational Operator : RelationalOperator  OutDataTypeStr=boolean  RndMeth=Simplest
  counter : DiscreteIntegrator  ExternalReset=either  SampleTime=-1  LimitOutput=on  UpperSaturationLimit=10  LowerSaturationLimit=-10  ICPrevOutput=DiscIntNeverNeededParam  ICPrevScaledInput=DiscIntNeverNeededParam
  DSLow2MidDistractn : Outport
  wires:
  Relational Operator/1 -> DSLow2MidDistractn/1
  Compare To Constant8/1 -> Logical Operator/5
  Compare To Constant4/1 -> Logical Operator/4
  Compare To Constant2/1 -> Logical Operator/3
  Compare To Constant/1 -> Logical Operator/1
  Compare To Constant1/1 -> Logical Operator/2
  canDistrctnQlty/1 -> Compare To Constant4/1, Compare To Constant8/1
  Logical Operator/1 -> Data Type Conversion/1
  canDistrctnLevel/1 -> Compare To Constant2/1
  canHeadDetn/1 -> Compare To Constant1/1
  canDMSSts/1 -> Compare To Constant/1
  PtDSLow2MidDistractn/1 -> Relational Operator/2
  counter/1 -> Relational Operator/1
  Data Type Conversion/1 -> counter/2, counter/1

== system Noa_Nofusion_backup/Common/Subsystem7/DS/DriverStsConditnJudge/DSLow2MidDrowsnsJudge ==
  note: %Note
      | Conditions of drowsns state from Low to Middle as follow:
      | DMSSts_ACC is 0x02: Active
      | && HeadDetn is 0x01: Yes
      | && DrowsnsLevel_ACC is 0x2: Middle level Drowsiness
      | && DrowsnsQlty_ACC≥85%
      | && During time≥3s(adjustable)
  canDMSSts : Inport
  canHeadDetn : Inport  Port=2
  canDrowsnsLevel : Inport  Port=3
  PtDSLow2MidDrowsns : Inport  Port=4
  Compare To Constant : simulink/Logic and Bit Operations/Compare To Constant  relop===  const=2  OutDataTypeStr=boolean
  Compare To Constant1 : simulink/Logic and Bit Operations/Compare To Constant  relop===  const=1  OutDataTypeStr=boolean
  Compare To Constant2 : simulink/Logic and Bit Operations/Compare To Constant  relop===  const=2  OutDataTypeStr=boolean
  Data Type Conversion : DataTypeConversion  OutDataTypeStr=single
  Logical Operator : Logic  Inputs=3  AllPortsSameDT=off  OutDataTypeStr=boolean
  Relational Operator : RelationalOperator  OutDataTypeStr=boolean  RndMeth=Simplest
  counter : DiscreteIntegrator  ExternalReset=either  SampleTime=-1  LimitOutput=on  UpperSaturationLimit=10  LowerSaturationLimit=-10  ICPrevOutput=DiscIntNeverNeededParam  ICPrevScaledInput=DiscIntNeverNeededParam
  DSLow2MidDrowsns : Outport
  wires:
  canDMSSts/1 -> Compare To Constant/1
  canHeadDetn/1 -> Compare To Constant1/1
  canDrowsnsLevel/1 -> Compare To Constant2/1
  Logical Operator/1 -> Data Type Conversion/1
  counter/1 -> Relational Operator/1
  Compare To Constant1/1 -> Logical Operator/2
  Compare To Constant/1 -> Logical Operator/1
  Compare To Constant2/1 -> Logical Operator/3
  Relational Operator/1 -> DSLow2MidDrowsns/1
  PtDSLow2MidDrowsns/1 -> Relational Operator/2
  Data Type Conversion/1 -> counter/2, counter/1

== system Noa_Nofusion_backup/Common/Subsystem7/DS/DriverStsConditnJudge/DSMidHi1Hi22LowDistractnJudge ==
  note: %Note
      | Conditions of distraction state from Middle∥High Level 1∥High Level 2 to Low as follow:
      | DMSSts_ACC is 0x02: Active
      | && HeadDetn is 0x01: Yes
      | && DistrctnLevel_ACC is 0x01: Low level distraction
      | && DistrctnQlty_ACC≥ 85%
      | && During time≥0.5s(adjustable)
  canDMSSts : Inport
  canHeadDetn : Inport  Port=2
  canDistrctnLevel : Inport  Port=3
  canDistrctnQlty : Inport  Port=4
  Compare To Constant : simulink/Logic and Bit Operations/Compare To Constant  relop===  const=2  OutDataTypeStr=boolean
  Compare To Constant1 : simulink/Logic and Bit Operations/Compare To Constant  relop===  const=1  OutDataTypeStr=boolean
  Compare To Constant2 : simulink/Logic and Bit Operations/Compare To Constant  relop===  const=1  OutDataTypeStr=boolean
  Compare To Constant4 : simulink/Logic and Bit Operations/Compare To Constant  relop=>=  const=85  OutDataTypeStr=boolean
  Compare To Constant5 : simulink/Logic and Bit Operations/Compare To Constant  relop=>=  const=0.5  OutDataTypeStr=boolean
  Compare To Constant8 : simulink/Logic and Bit Operations/Compare To Constant  relop=<=  const=100  OutDataTypeStr=boolean
  Data Type Conversion : DataTypeConversion  OutDataTypeStr=single
  Logical Operator : Logic  Inputs=5  AllPortsSameDT=off  OutDataTypeStr=boolean
  counter : DiscreteIntegrator  ExternalReset=either  SampleTime=-1  LimitOutput=on  UpperSaturationLimit=10  LowerSaturationLimit=-10  ICPrevOutput=DiscIntNeverNeededParam  ICPrevScaledInput=DiscIntNeverNeededParam
  DSMidHi1Hi22LowDistractn : Outport
  wires:
  Compare To Constant5/1 -> DSMidHi1Hi22LowDistractn/1
  Compare To Constant8/1 -> Logical Operator/5
  Compare To Constant4/1 -> Logical Operator/4
  Compare To Constant2/1 -> Logical Operator/3
  Compare To Constant/1 -> Logical Operator/1
  Compare To Constant1/1 -> Logical Operator/2
  canDistrctnQlty/1 -> Compare To Constant4/1, Compare To Constant8/1
  Logical Operator/1 -> Data Type Conversion/1
  canDistrctnLevel/1 -> Compare To Constant2/1
  canHeadDetn/1 -> Compare To Constant1/1
  canDMSSts/1 -> Compare To Constant/1
  counter/1 -> Compare To Constant5/1
  Data Type Conversion/1 -> counter/2, counter/1

== system Noa_Nofusion_backup/Common/Subsystem7/DS/DriverStsConditnJudge/DSMidHi1Hi22LowDrowsnsJudge ==
  note: %Note
      | Conditions of drowsns state from Middle∥High Level 1∥High Level 2 to Low as follow:
      | DMSSts_ACC is 0x02: Active
      | && HeadDetn is 0x01: Yes
      | && DrowsnsLevel_ACC is 0x1: Low level Drowsiness
      | && DrowsnsQlty_ACC≥85%
      | && During time≥0.5s(adjustable)
  canDMSSts : Inport
  canHeadDetn : Inport  Port=2
  canDrowsnsLevel : Inport  Port=3
  Compare To Constant : simulink/Logic and Bit Operations/Compare To Constant  relop===  const=2  OutDataTypeStr=boolean
  Compare To Constant1 : simulink/Logic and Bit Operations/Compare To Constant  relop===  const=1  OutDataTypeStr=boolean
  Compare To Constant2 : simulink/Logic and Bit Operations/Compare To Constant  relop===  const=1  OutDataTypeStr=boolean
  Compare To Constant5 : simulink/Logic and Bit Operations/Compare To Constant  relop=>=  const=0.5  OutDataTypeStr=boolean
  Data Type Conversion : DataTypeConversion  OutDataTypeStr=single
  Logical Operator : Logic  Inputs=3  AllPortsSameDT=off  OutDataTypeStr=boolean
  counter : DiscreteIntegrator  ExternalReset=either  SampleTime=-1  LimitOutput=on  UpperSaturationLimit=10  LowerSaturationLimit=-10  ICPrevOutput=DiscIntNeverNeededParam  ICPrevScaledInput=DiscIntNeverNeededParam
  DSMidHi1Hi22LowDrowsns : Outport
  wires:
  canDMSSts/1 -> Compare To Constant/1
  canHeadDetn/1 -> Compare To Constant1/1
  canDrowsnsLevel/1 -> Compare To Constant2/1
  Logical Operator/1 -> Data Type Conversion/1
  Compare To Constant1/1 -> Logical Operator/2
  Compare To Constant/1 -> Logical Operator/1
  Compare To Constant2/1 -> Logical Operator/3
  Compare To Constant5/1 -> DSMidHi1Hi22LowDrowsns/1
  counter/1 -> Compare To Constant5/1
  Data Type Conversion/1 -> counter/2, counter/1

== system Noa_Nofusion_backup/Common/Subsystem7/DS/DriverStsConditnJudge/DSMidHi1Hi22NoDistractnJudge ==
  note: %Note
      | In order to cover one case at which distraction is no distraction but drowsns is low/middle/high 1/high2,add this
      | transition from low/middle/high 1/high2 distraction to no distraction.Conditions as follow:
      | DMSSts_ACC is 0x02: Active
      | && HeadDetn is 0x01: Yes
      | && DistrctnLevel_ACC is 0x00: No distraction
      | && DistrctnQlty_ACC≥ 85%
      | && During time is same as time of other to good
  canDMSSts : Inport
  canHeadDetn : Inport  Port=2
  canDistrctnLevel : Inport  Port=3
  canDistrctnQlty : Inport  Port=4
  Compare To Constant : simulink/Logic and Bit Operations/Compare To Constant  relop===  const=2  OutDataTypeStr=boolean
  Compare To Constant1 : simulink/Logic and Bit Operations/Compare To Constant  relop===  const=1  OutDataTypeStr=boolean
  Compare To Constant2 : simulink/Logic and Bit Operations/Compare To Constant  relop===  const=0  OutDataTypeStr=boolean
  Compare To Constant4 : simulink/Logic and Bit Operations/Compare To Constant  relop=>=  const=85  OutDataTypeStr=boolean
  Compare To Constant5 : simulink/Logic and Bit Operations/Compare To Constant  relop=>=  const=0.5  OutDataTypeStr=boolean
  Compare To Constant8 : simulink/Logic and Bit Operations/Compare To Constant  relop=<=  const=100  OutDataTypeStr=boolean
  Data Type Conversion : DataTypeConversion  OutDataTypeStr=single
  Logical Operator : Logic  Inputs=5  AllPortsSameDT=off  OutDataTypeStr=boolean
  counter : DiscreteIntegrator  ExternalReset=either  SampleTime=-1  LimitOutput=on  UpperSaturationLimit=10  LowerSaturationLimit=-10  ICPrevOutput=DiscIntNeverNeededParam  ICPrevScaledInput=DiscIntNeverNeededParam
  DSMidHi1Hi22NoDistractn : Outport
  wires:
  Compare To Constant5/1 -> DSMidHi1Hi22NoDistractn/1
  Compare To Constant8/1 -> Logical Operator/5
  Compare To Constant4/1 -> Logical Operator/4
  Compare To Constant2/1 -> Logical Operator/3
  Compare To Constant/1 -> Logical Operator/1
  Compare To Constant1/1 -> Logical Operator/2
  canDistrctnQlty/1 -> Compare To Constant4/1, Compare To Constant8/1
  counter/1 -> Compare To Constant5/1
  Logical Operator/1 -> Data Type Conversion/1
  canDistrctnLevel/1 -> Compare To Constant2/1
  canHeadDetn/1 -> Compare To Constant1/1
  canDMSSts/1 -> Compare To Constant/1
  Data Type Conversion/1 -> counter/2, counter/1

== system Noa_Nofusion_backup/Common/Subsystem7/DS/DriverStsConditnJudge/DSMidHi1Hi22NoDrowsnsJudge ==
  note: %Note
      | In order to cover one case at which drowsns is no drowsiness but distraction is low/middle/high 1/high2,add this
      | transition from low/middle/high 1/high2 drowsiness to no drowsiness.Conditions as follow:
      | DMSSts_ACC is 0x02: Active
      | && HeadDetn is 0x01: Yes
      | && DrowsnsLevel_ACC is：0x0: No Drowsiness
      | && DrowsnsQlty_ACC≥85%
      | && During time is same as time of other to good
  canDMSSts : Inport
  canHeadDetn : Inport  Port=2
  canDrowsnsLevel : Inport  Port=3
  Compare To Constant : simulink/Logic and Bit Operations/Compare To Constant  relop===  const=2  OutDataTypeStr=boolean
  Compare To Constant1 : simulink/Logic and Bit Operations/Compare To Constant  relop===  const=1  OutDataTypeStr=boolean
  Compare To Constant2 : simulink/Logic and Bit Operations/Compare To Constant  relop===  const=0  OutDataTypeStr=boolean
  Compare To Constant5 : simulink/Logic and Bit Operations/Compare To Constant  relop=>=  const=0.5  OutDataTypeStr=boolean
  Data Type Conversion : DataTypeConversion  OutDataTypeStr=single
  Logical Operator : Logic  Inputs=3  AllPortsSameDT=off  OutDataTypeStr=boolean
  counter : DiscreteIntegrator  ExternalReset=either  SampleTime=-1  LimitOutput=on  UpperSaturationLimit=10  LowerSaturationLimit=-10  ICPrevOutput=DiscIntNeverNeededParam  ICPrevScaledInput=DiscIntNeverNeededParam
  DSMidHi1Hi22NoDrowsns : Outport
  wires:
  canDMSSts/1 -> Compare To Constant/1
  canHeadDetn/1 -> Compare To Constant1/1
  canDrowsnsLevel/1 -> Compare To Constant2/1
  Logical Operator/1 -> Data Type Conversion/1
  counter/1 -> Compare To Constant5/1
  Compare To Constant1/1 -> Logical Operator/2
  Compare To Constant/1 -> Logical Operator/1
  Compare To Constant2/1 -> Logical Operator/3
  Compare To Constant5/1 -> DSMidHi1Hi22NoDrowsns/1
  Data Type Conversion/1 -> counter/2, counter/1

== system Noa_Nofusion_backup/Common/Subsystem7/DS/DriverStsConditnJudge/DSOther2GoodJudge ==
  note: %Note
      | Conditions of distraction state from Unbelievable∥Low∥Middle∥High Level 1∥High Level 2 to Good as follows:
      | DMSSts_ACC is 0x02: Active
      | && HeadDetn is 0x01: Yes
      | && DistrctnLevel_ACC is 0x00: No distraction
      | && DistrctnQlty_ACC≥ 85%
      | && DrowsnsLevel_ACC is：0x0: No Drowsiness
      | && DrowsnsQlty_ACC≥85%
      | && During time≥0.5s
  canDMSSts : Inport
  canHeadDetn : Inport  Port=2
  canDistrctnLevel : Inport  Port=3
  canDistrctnQlty : Inport  Port=4
  canDrowsnsLevel : Inport  Port=5
  Compare To Constant : simulink/Logic and Bit Operations/Compare To Constant  relop===  const=2  OutDataTypeStr=boolean
  Compare To Constant1 : simulink/Logic and Bit Operations/Compare To Constant  relop===  const=1  OutDataTypeStr=boolean
  Compare To Constant2 : simulink/Logic and Bit Operations/Compare To Constant  relop===  const=0  OutDataTypeStr=boolean
  Compare To Constant3 : simulink/Logic and Bit Operations/Compare To Constant  relop=>=  const=85  OutDataTypeStr=boolean
  Compare To Constant4 : simulink/Logic and Bit Operations/Compare To Constant  relop=<=  const=100  OutDataTypeStr=boolean
  Compare To Constant5 : simulink/Logic and Bit Operations/Compare To Constant  relop=>=  const=0.5  OutDataTypeStr=boolean
  Compare To Constant6 : simulink/Logic and Bit Operations/Compare To Constant  relop===  const=0  OutDataTypeStr=boolean
  Data Type Conversion : DataTypeConversion  OutDataTypeStr=single
  Logical Operator : Logic  Inputs=6  AllPortsSameDT=off  OutDataTypeStr=boolean
  counter : DiscreteIntegrator  ExternalReset=either  SampleTime=-1  LimitOutput=on  UpperSaturationLimit=10  LowerSaturationLimit=-10  ICPrevOutput=DiscIntNeverNeededParam  ICPrevScaledInput=DiscIntNeverNeededParam
  DSOther2Good : Outport
  wires:
  canDMSSts/1 -> Compare To Constant/1
  canHeadDetn/1 -> Compare To Constant1/1
  canDistrctnLevel/1 -> Compare To Constant2/1
  canDistrctnQlty/1 -> Compare To Constant4/1, Compare To Constant3/1
  Logical Operator/1 -> Data Type Conversion/1
  counter/1 -> Compare To Constant5/1
  canDrowsnsLevel/1 -> Compare To Constant6/1
  Compare To Constant/1 -> Logical Operator/1
  Compare To Constant1/1 -> Logical Operator/2
  Compare To Constant2/1 -> Logical Operator/3
  Compare To Constant3/1 -> Logical Operator/4
  Compare To Constant4/1 -> Logical Operator/5
  Compare To Constant6/1 -> Logical Operator/6
  Compare To Constant5/1 -> DSOther2Good/1
  Data Type Conversion/1 -> counter/2, counter/1

== system Noa_Nofusion_backup/Common/Subsystem7/DS/DriverStsConditnJudge/DSOther2Hi1DistractnJudge ==
  note: %Note
      | Conditions of distraction state from other state to High 1 as follow:
      | DMSSts_ACC is 0x02: Active
      | && HeadDetn is 0x01: Yes
      | && DistrctnLevel_ACC is 0x03: Hi level distraction
      | && DistrctnQlty_ACC≥ 85%
      | && During time≥2s(adjustable)
  canDMSSts : Inport
  canHeadDetn : Inport  Port=2
  canDistrctnLevel : Inport  Port=3
  canDistrctnQlty : Inport  Port=4
  PtDSOther2Hi1Distractn : Inport  Port=5
  Compare To Constant : simulink/Logic and Bit Operations/Compare To Constant  relop===  const=2  OutDataTypeStr=boolean
  Compare To Constant1 : simulink/Logic and Bit Operations/Compare To Constant  relop===  const=1  OutDataTypeStr=boolean
  Compare To Constant2 : simulink/Logic and Bit Operations/Compare To Constant  relop===  const=3  OutDataTypeStr=boolean
  Compare To Constant4 : simulink/Logic and Bit Operations/Compare To Constant  relop=>=  const=85  OutDataTypeStr=boolean
  Compare To Constant8 : simulink/Logic and Bit Operations/Compare To Constant  relop=<=  const=100  OutDataTypeStr=boolean
  Data Type Conversion : DataTypeConversion  OutDataTypeStr=single
  Logical Operator : Logic  Inputs=5  AllPortsSameDT=off  OutDataTypeStr=boolean
  Relational Operator : RelationalOperator  OutDataTypeStr=boolean  RndMeth=Simplest
  counter : DiscreteIntegrator  ExternalReset=either  SampleTime=-1  LimitOutput=on  UpperSaturationLimit=10  LowerSaturationLimit=-10  ICPrevOutput=DiscIntNeverNeededParam  ICPrevScaledInput=DiscIntNeverNeededParam
  DSOther2Hi1Distractn : Outport
  wires:
  Logical Operator/1 -> Data Type Conversion/1
  canDMSSts/1 -> Compare To Constant/1
  canHeadDetn/1 -> Compare To Constant1/1
  canDistrctnLevel/1 -> Compare To Constant2/1
  canDistrctnQlty/1 -> Compare To Constant8/1, Compare To Constant4/1
  Compare To Constant1/1 -> Logical Operator/2
  Compare To Constant/1 -> Logical Operator/1
  Compare To Constant2/1 -> Logical Operator/3
  Compare To Constant4/1 -> Logical Operator/4
  Compare To Constant8/1 -> Logical Operator/5
  Relational Operator/1 -> DSOther2Hi1Distractn/1
  counter/1 -> Relational Operator/1
  PtDSOther2Hi1Distractn/1 -> Relational Operator/2
  Data Type Conversion/1 -> counter/2, counter/1
